simulink library "vehicle_dynamics_lib"  (R2012b)
settings: Solver=ode45  StartTime=0.0  StopTime=10.0  RelTol=1e-3
undefined symbols (not defined in the file): X, Y
settings Model: Creator=vismso  LastModifiedBy=vikafla

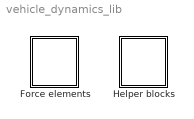
== system vehicle_dynamics_lib ==
  Force elements : Subsystem
  Helper blocks : Subsystem

== system vehicle_dynamics_lib/Force elements ==
  Spring-Damper : Subsystem  mask{dtype=Active, pdamp=on, c=[-1 1;-60.8e3 60.8e3], l0=0.253, d=[-1 1;-1.2e3 1.2e3], d_s_max=1200}
      mask prompts: dtype "Damper type"; pdamp "With passive damper?"; c "Spring stiffness table [displacement ...;force ...]"; l0 "Spring free length [m]"; d "Damper cushioning table [velocity ...;force ...]"; d_s_max "Maximum active damper damping value [Ns/m]"
      settings: MinAlgLoopOccurrences=on
      mask TypeOptions dtype: Semi-active | Active | Passive
      mask Callback dtype:
      | % set control visibilities
      | pdamp = get_param(gcb,'pdamp');
      | if strcmpi(get_param(gcb,'dtype'),'active')
      |     set_param(gcb,'MaskVisibilities',{'on','on','on','on',pdamp,'off'});
      |     set_param(gcb,'pdamp',pdamp);
      | elseif strcmpi(get_param(gcb,'dtype'),'passive')
      |     set_param(gcb,'MaskVisibilities',{'on','off','on','on','on','off'});
      |     set_param(gcb,'pdamp','on');
      | else
      |     set_param(gcb,'MaskVisibilities',{'on','off','on','on','off','on'});
      |     set_param(gcb,'pdamp','off');
      | end
      mask Callback pdamp:
      | tempvis = get_param(gcb,'MaskVisibilities');
      | if strcmpi(get_param(gcb,'pdamp'),'on')
      |     tempvis{5} = 'on';
      |     set_param(gcb,'MaskVisibilities',tempvis);
      | else
      |     tempvis{5} = 'off';
      |     set_param(gcb,'MaskVisibilities',tempvis);
      | end
      mask Display:
      | image(imread('damper.jpg'))
      | color('white')
      | port_label('input',2,'Actuator Force')
  Wheel forces & torques : Subsystem  mask{c=200e3, d=1e3, r0=0.24}
      mask prompts: c "Tire spring stiffness [N/m]"; d "Tire damper cushioning [N/(m/s)]"; r0 "Unloaded tire radius [m]"
      settings: MinAlgLoopOccurrences=on
      mask Display: image(imread('tire.jpg'))
  Wheel forces & torques (Pacejka stationary) : Subsystem  mask{c=200e3, d=1e3, r0=0.33, a=[1.799,0,1088,1140,6.026,0,-0.3589,1,0,-6.111e-3,-3.224e-2,0,0,0,0], b=[1.45,0,1088,0,129,0,0,0,-7,0,0]}
      mask prompts: c "Tire spring stiffness [N/m]"; d "Tire damper cushioning [N/(m/s)]"; r0 "Unloaded tire radius [m]"; a "Pacejka lateral a values (14)"; b "Pacejka longitudunal b values (10)"
      settings: MinAlgLoopOccurrences=on
      mask Display: image(imread('tire.jpg'))
  Wheel forces & torques (Pacejka transient) : Subsystem  mask{c=200e3, d=1e3, r0=0.33, a=[1.799,0,1088,1140,6.026,0,-0.3589,1,0,-6.111e-3,-3.224e-2,0,0,0,0], b=[1.45,0,1088,0,129,0,0,0,-7,0,0], Lx=0.2, Ly=0.2, Vlow=2}
      mask prompts: c "Tire spring stiffness [N/m]"; d "Tire damper cushioning [N/(m/s)]"; r0 "Unloaded tire radius [m]"; a "Pacejka lateral a values (15)"; b "Pacejka longitudunal b values (11)"; Lx "Longitudinal relaxation length [m]"; Ly "Lateral relaxation length [m]"; Vlow "Lower speed limit for slip damping [m/s]"
      settings: MinAlgLoopOccurrences=on
      mask Display: image(imread('tire.jpg'))

== system vehicle_dynamics_lib/Helper blocks ==
  2nd order butterworth high-pass : Subsystem  mask{wf=0.07, zeta=1/sqrt(2)}
      mask prompts: wf "Cut-off frequency [Hz]"; zeta "Damping coefficient"
      mask init:
      | x = 0:1:2;
      | y = [0;1;1];
      mask Display:
      | plot(x,y)
      | text(1,0.5,'HP')
  Lookup-table for ground geometry : Subsystem  mask(Lookup-table for ground geometry){}
      mask help:
      | This block contains the lookup tables holding data for the ground grid
      | lookup. It reads the variables X, Y, Z ,Nx , Ny, Nz from Matlabs
      | workspace. All of these variables must be meshgrids of equal size.
      |
      | X,Y - X,Y Positions
      | Z - Grid of ground height corresponding to X,Y values
      | Nx,Ny,Nz - Components of normal vector for each X,Y point of the ground
      |
      | Given input x,y coordinates, the block outputs the corresponding ground
      | height Z value and the points surface normal.
  Numerical differentiator : Subsystem  mask{Ts=0.01}
      mask prompts: Ts "First order lag time constant [s]"
      mask init:
      | x = 0:0.1:9;
      | y = exp(-x);
      mask Display:
      | plot(x,y)
      | text(3.5,0.5,'d/dt')
  "q1dot -> q" : Subsystem  mask(Euler angle -> Quaternion integration){}
      mask help:
      | This block internally integrates given euler angles as quaternions, thus
      | evading gimbal lock.
      mask Display: droots([],[0],1)

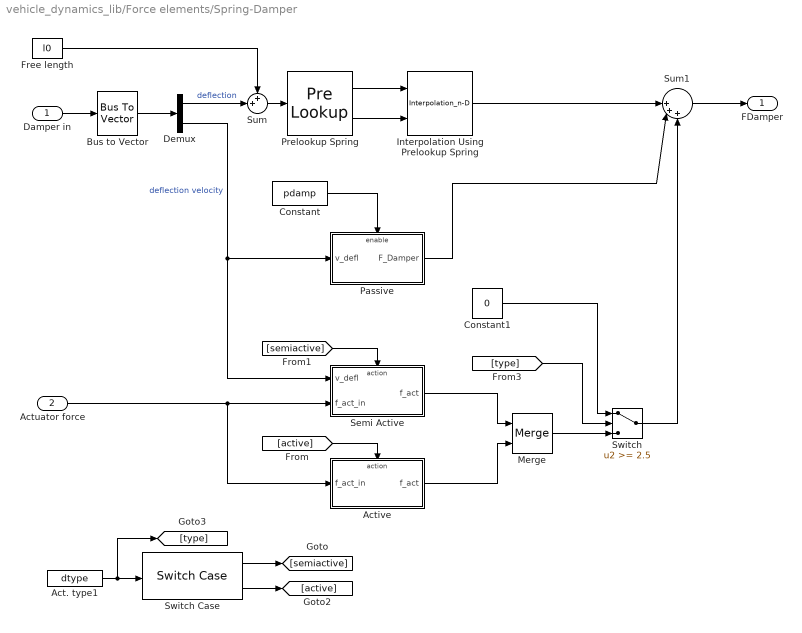
== system vehicle_dynamics_lib/Force elements/Spring-Damper ==
  Damper in : Inport
  Actuator force : Inport  Port=2
  Act. type1 : Constant  Value=dtype
      settings: AttributesFormatString=1 = semi-active\n2 = active\n3 = passive
  Active : Subsystem  TreatAsAtomicUnit=on
  Bus to Vector : BusToVector
  Constant : Constant  Value=pdamp
  Constant1 : Constant  Value=0
  Demux : Demux  Outputs=2
  Free length : Constant  Value=l0
  Interpolation Using Prelookup Spring : Interpolation_n-D  NumberOfTableDimensions=1  Table=c(2,:)
      settings: InputPortMap=u0,u1
  Merge : Merge
  Passive : Subsystem  TreatAsAtomicUnit=on
  Prelookup Spring : PreLookup  BreakpointsData=c(1,:)  ExtrapMethod=Linear
  Semi Active : Subsystem  TreatAsAtomicUnit=on
  Sum : Sum  Inputs=++|
  Sum1 : Sum  Inputs=||+++
  Switch : Switch  Threshold=2.5
  Switch Case : SwitchCase  CaseConditions={1,2}  ShowDefaultCase=off
  FDamper : Outport
  wires:
  Demux/2 -> Passive/1(v_defl), Semi Active/1(v_defl)  "deflection velocity"
  Demux/1 -> Sum/2  "deflection"
  Bus to Vector/1 -> Demux/1
  Interpolation Using Prelookup Spring/1 -> Sum1/1
  Sum1/1 -> FDamper/1
  Free length/1 -> Sum/1
  Damper in/1 -> Bus to Vector/1
  Sum/1 -> Prelookup Spring/1
  Prelookup Spring/2 -> Interpolation Using Prelookup Spring/2
  Prelookup Spring/1 -> Interpolation Using Prelookup Spring/1
  Act. type1/1 -> Switch Case/1, [type]
  Actuator force/1 -> Semi Active/2(f_act_in), Active/1(f_act_in)
  Switch Case/1 -> [semiactive]
  Switch Case/2 -> [active]
  [active] -> Active/Action
  [semiactive] -> Semi Active/Action
  [type] -> Switch/2
  Constant/1 -> Passive/Enable
  Passive/1(F_Damper) -> Sum1/2
  Active/1(f_act) -> Merge/2
  Semi Active/1(f_act) -> Merge/1
  Switch/1 -> Sum1/3
  Constant1/1 -> Switch/1
  Merge/1 -> Switch/3

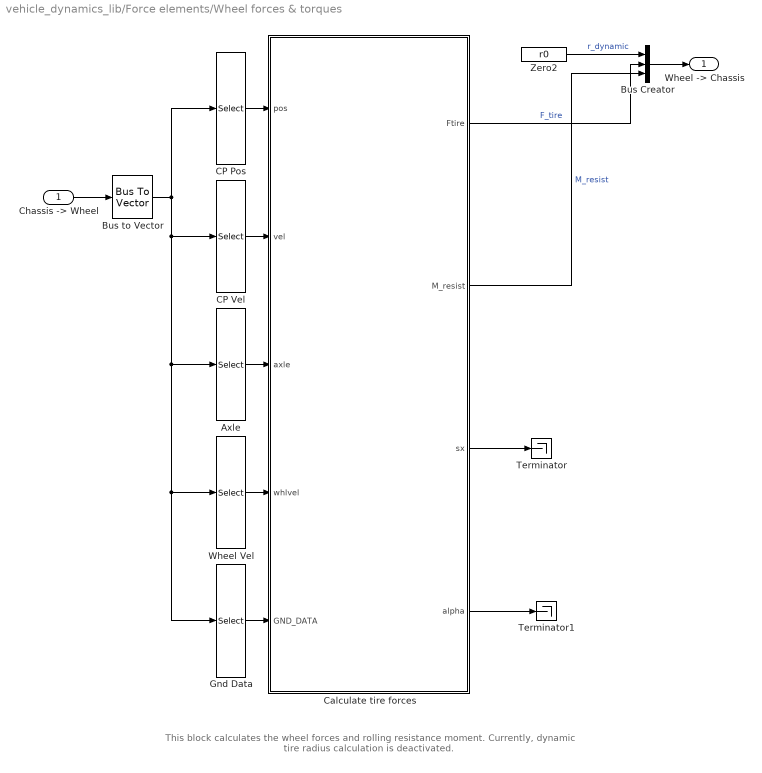
== system vehicle_dynamics_lib/Force elements/Wheel forces & torques ==
  note: This block calculates the wheel forces and rolling resistance moment.
      | Currently, dynamic tire radius calculation is deactivated.
  "Chassis -> Wheel" : Inport
  Axle : Selector  InputPortWidth=16  IndexOptions=Index vector (dialog)  Indices=[1:3]  OutputSizes=1
  Bus Creator : BusCreator  Inputs=3
  Bus to Vector : BusToVector
  CP Pos : Selector  InputPortWidth=16  IndexOptions=Index vector (dialog)  Indices=[4:6]  OutputSizes=1
  CP Vel : Selector  InputPortWidth=16  IndexOptions=Index vector (dialog)  Indices=[7:9]  OutputSizes=1
  Calculate tire forces : MATLAB Function  TreatAsAtomicUnit=on
  Gnd Data : Selector  InputPortWidth=16  IndexOptions=Index vector (dialog)  Indices=[13:16]  OutputSizes=1
  Terminator : Terminator
  Terminator1 : Terminator
  Wheel Vel : Selector  InputPortWidth=16  IndexOptions=Index vector (dialog)  Indices=[10:12]  OutputSizes=1
  Zero2 : Constant  Value=r0
  "Wheel -> Chassis" : Outport
  wires:
  Gnd Data/1 -> Calculate tire forces/5(GND_DATA)
  Calculate tire forces/4(alpha) -> Terminator1/1
  Calculate tire forces/3(sx) -> Terminator/1
  Bus Creator/1 -> "Wheel -> Chassis"/1
  Calculate tire forces/2(M_resist) -> Bus Creator/3  "M_resist"
  Zero2/1 -> Bus Creator/1  "r_dynamic"
  CP Pos/1 -> Calculate tire forces/1(pos)
  CP Vel/1 -> Calculate tire forces/2(vel)
  Calculate tire forces/1(Ftire) -> Bus Creator/2  "F_tire"
  "Chassis -> Wheel"/1 -> Bus to Vector/1
  Bus to Vector/1 -> CP Pos/1, CP Vel/1, Gnd Data/1, Wheel Vel/1, Axle/1
  Axle/1 -> Calculate tire forces/3(axle)
  Wheel Vel/1 -> Calculate tire forces/4(whlvel)

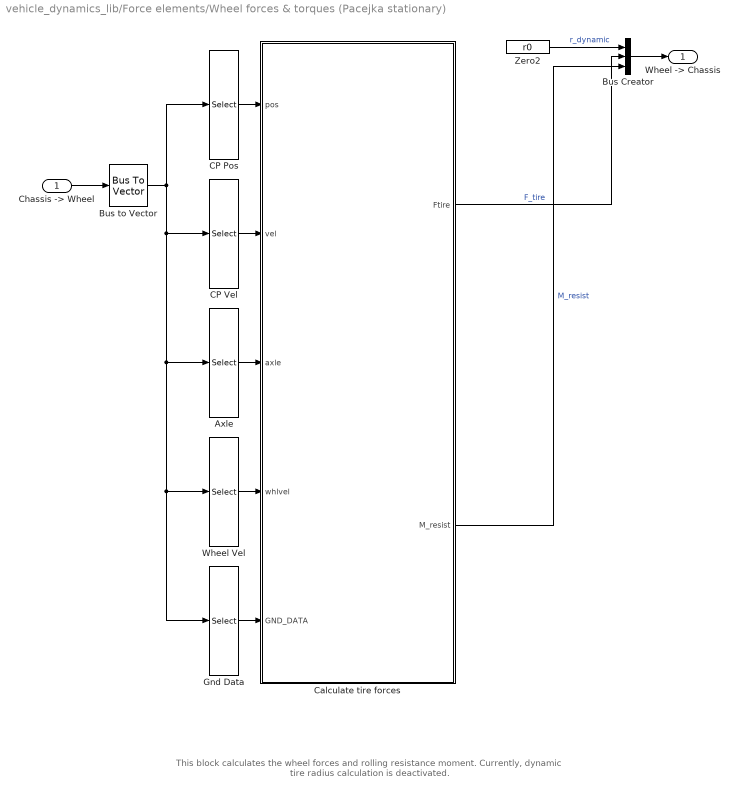
== system vehicle_dynamics_lib/Force elements/Wheel forces & torques (Pacejka stationary) ==
  note: This block calculates the wheel forces and rolling resistance moment.
      | Currently, dynamic tire radius calculation is deactivated.
  "Chassis -> Wheel" : Inport
  Axle : Selector  InputPortWidth=16  IndexOptions=Index vector (dialog)  Indices=[1:3]  OutputSizes=1
  Bus Creator : BusCreator  Inputs=3
  Bus to Vector : BusToVector
  CP Pos : Selector  InputPortWidth=16  IndexOptions=Index vector (dialog)  Indices=[4:6]  OutputSizes=1
  CP Vel : Selector  InputPortWidth=16  IndexOptions=Index vector (dialog)  Indices=[7:9]  OutputSizes=1
  Calculate tire forces : MATLAB Function  TreatAsAtomicUnit=on
  Gnd Data : Selector  InputPortWidth=16  IndexOptions=Index vector (dialog)  Indices=[13:16]  OutputSizes=1
  Wheel Vel : Selector  InputPortWidth=16  IndexOptions=Index vector (dialog)  Indices=[10:12]  OutputSizes=1
  Zero2 : Constant  Value=r0
  "Wheel -> Chassis" : Outport
  wires:
  Gnd Data/1 -> Calculate tire forces/5(GND_DATA)
  Bus Creator/1 -> "Wheel -> Chassis"/1
  Calculate tire forces/2(M_resist) -> Bus Creator/3  "M_resist"
  Zero2/1 -> Bus Creator/1  "r_dynamic"
  CP Pos/1 -> Calculate tire forces/1(pos)
  CP Vel/1 -> Calculate tire forces/2(vel)
  Calculate tire forces/1(Ftire) -> Bus Creator/2  "F_tire"
  "Chassis -> Wheel"/1 -> Bus to Vector/1
  Bus to Vector/1 -> CP Pos/1, CP Vel/1, Gnd Data/1, Wheel Vel/1, Axle/1
  Axle/1 -> Calculate tire forces/3(axle)
  Wheel Vel/1 -> Calculate tire forces/4(whlvel)

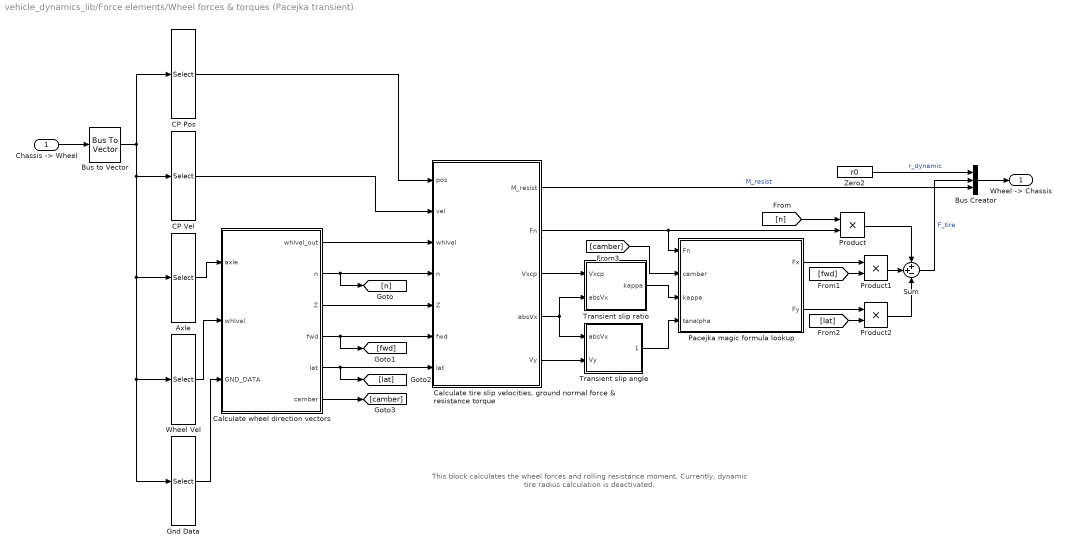
== system vehicle_dynamics_lib/Force elements/Wheel forces & torques (Pacejka transient) ==
  note: This block calculates the wheel forces and rolling resistance moment.
      | Currently, dynamic tire radius calculation is deactivated.
  "Chassis -> Wheel" : Inport
  Axle : Selector  InputPortWidth=16  IndexOptions=Index vector (dialog)  Indices=[1:3]  OutputSizes=1
  Bus Creator : BusCreator  Inputs=3
  Bus to Vector : BusToVector
  CP Pos : Selector  InputPortWidth=16  IndexOptions=Index vector (dialog)  Indices=[4:6]  OutputSizes=1
  CP Vel : Selector  InputPortWidth=16  IndexOptions=Index vector (dialog)  Indices=[7:9]  OutputSizes=1
  "Calculate tire slip velocities, ground normal force & resistance torque" : MATLAB Function  TreatAsAtomicUnit=on
  Calculate wheel direction vectors : MATLAB Function  TreatAsAtomicUnit=on
  Gnd Data : Selector  InputPortWidth=16  IndexOptions=Index vector (dialog)  Indices=[13:16]  OutputSizes=1
  Pacejka magic formula lookup : MATLAB Function  TreatAsAtomicUnit=on
  Product : Product  RndMeth=Zero
  Product1 : Product  RndMeth=Zero
  Product2 : Product  RndMeth=Zero
  Sum : Sum  Inputs=++-
  Transient slip angle : Subsystem
  Transient slip ratio : Subsystem
  Wheel Vel : Selector  InputPortWidth=16  IndexOptions=Index vector (dialog)  Indices=[10:12]  OutputSizes=1
  Zero2 : Constant  Value=r0
  "Wheel -> Chassis" : Outport
  wires:
  Bus to Vector/1 -> Axle/1, Wheel Vel/1, Gnd Data/1, CP Vel/1, CP Pos/1
  "Chassis -> Wheel"/1 -> Bus to Vector/1
  Sum/1 -> Bus Creator/2  "F_tire"
  CP Pos/1 -> "Calculate tire slip velocities, ground normal force & resistance torque"/1(pos)
  Zero2/1 -> Bus Creator/1  "r_dynamic"
  Bus Creator/1 -> "Wheel -> Chassis"/1
  CP Vel/1 -> "Calculate tire slip velocities, ground normal force & resistance torque"/2(vel)
  "Calculate tire slip velocities, ground normal force & resistance torque"/3(Vxcp) -> Transient slip ratio/1(Vxcp)
  "Calculate tire slip velocities, ground normal force & resistance torque"/4(absVx) -> Transient slip ratio/2(absVx), Transient slip angle/1(absVx)
  "Calculate tire slip velocities, ground normal force & resistance torque"/5(Vy) -> Transient slip angle/2(Vy)
  "Calculate tire slip velocities, ground normal force & resistance torque"/2(Fn) -> Pacejka magic formula lookup/1(Fn), Product/2
  Transient slip ratio/1(kappa) -> Pacejka magic formula lookup/3(kappa)
  Transient slip angle/1(tanalpha) -> Pacejka magic formula lookup/4(tanalpha)
  Axle/1 -> Calculate wheel direction vectors/1(axle)
  Wheel Vel/1 -> Calculate wheel direction vectors/2(whlvel)
  Gnd Data/1 -> Calculate wheel direction vectors/3(GND_DATA)
  Calculate wheel direction vectors/2(n) -> "Calculate tire slip velocities, ground normal force & resistance torque"/4(n), [n]
  Calculate wheel direction vectors/3(Z) -> "Calculate tire slip velocities, ground normal force & resistance torque"/5(Z)
  Calculate wheel direction vectors/4(fwd) -> "Calculate tire slip velocities, ground normal force & resistance torque"/6(fwd), [fwd]
  Calculate wheel direction vectors/5(lat) -> "Calculate tire slip velocities, ground normal force & resistance torque"/7(lat), [lat]
  Calculate wheel direction vectors/1(whlvel_out) -> "Calculate tire slip velocities, ground normal force & resistance torque"/3(whlvel)
  "Calculate tire slip velocities, ground normal force & resistance torque"/1(M_resist) -> Bus Creator/3  "M_resist"
  Product/1 -> Sum/1
  [n] -> Product/1
  Product1/1 -> Sum/2
  Pacejka magic formula lookup/1(Fx) -> Product1/1
  [fwd] -> Product1/2
  Pacejka magic formula lookup/2(Fy) -> Product2/1
  [lat] -> Product2/2
  Product2/1 -> Sum/3
  Calculate wheel direction vectors/6(camber) -> [camber]
  [camber] -> Pacejka magic formula lookup/2(camber)

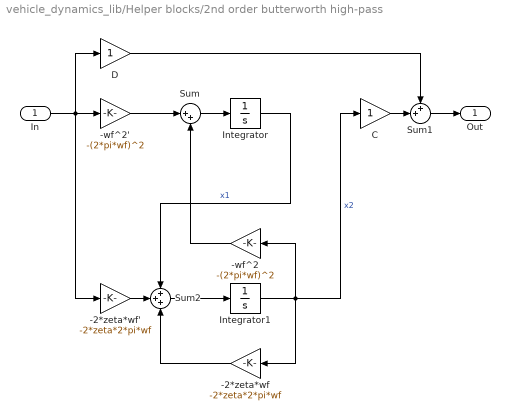
== system vehicle_dynamics_lib/Helper blocks/2nd order butterworth high-pass ==
  In : Inport
  -2*zeta*wf : Gain  Gain=-2*zeta*2*pi*wf
  -2*zeta*wf' : Gain  Gain=-2*zeta*2*pi*wf
  -wf^2 : Gain  Gain=-(2*pi*wf)^2
  -wf^2' : Gain  Gain=-(2*pi*wf)^2
  C : Gain
  D : Gain
  Integrator : Integrator
  Integrator1 : Integrator
  Sum : Sum  Inputs=|++
  Sum1 : Sum  Inputs=++|
  Sum2 : Sum  Inputs=+++
  Out : Outport
  wires:
  D/1 -> Sum1/1
  C/1 -> Sum1/2
  Integrator/1 -> Sum2/1  "x1"
  -wf^2'/1 -> Sum/1
  In/1 -> -wf^2'/1, D/1, -2*zeta*wf'/1
  Sum/1 -> Integrator/1
  Integrator1/1 -> -wf^2/1, -2*zeta*wf/1, C/1  "x2"
  Sum2/1 -> Integrator1/1
  -wf^2/1 -> Sum/2
  -2*zeta*wf/1 -> Sum2/3
  -2*zeta*wf'/1 -> Sum2/2
  Sum1/1 -> Out/1

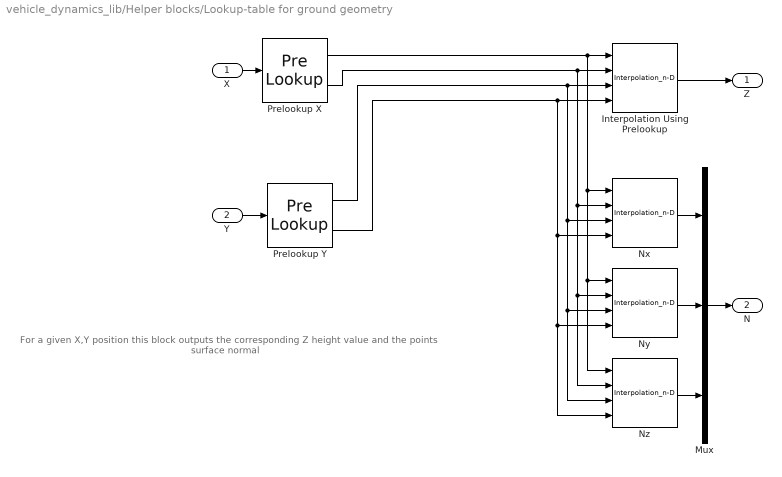
== system vehicle_dynamics_lib/Helper blocks/Lookup-table for ground geometry ==
  note: For a given X,Y position this block outputs the
      | corresponding Z height value and the points surface normal
  X : Inport
  Y : Inport  Port=2
  Interpolation Using Prelookup : Interpolation_n-D  Table=Z.'  RemoveProtectionIndex=on  TableDataTypeStr=Inherit: Inherit from 'Table data'
  Mux : Mux  Inputs=3
  Nx : Interpolation_n-D  Table=Nx.'  ExtrapMethod=Clip  RemoveProtectionIndex=on  TableDataTypeStr=Inherit: Inherit from 'Table data'
  Ny : Interpolation_n-D  Table=Ny.'  ExtrapMethod=Clip  RemoveProtectionIndex=on  TableDataTypeStr=Inherit: Inherit from 'Table data'
  Nz : Interpolation_n-D  Table=Nz.'  ExtrapMethod=Clip  RemoveProtectionIndex=on  TableDataTypeStr=Inherit: Inherit from 'Table data'
  Prelookup X : PreLookup  BreakpointsData=X(1,:)  ExtrapMethod=Linear  BreakpointDataTypeStr=Inherit: Inherit from 'Breakpoint data'
  Prelookup Y : PreLookup  BreakpointsData=Y(:,1)  ExtrapMethod=Linear  BreakpointDataTypeStr=Inherit: Inherit from 'Breakpoint data'
  Z : Outport
  N : Outport  Port=2  PortDimensions=3
  wires:
  Mux/1 -> N/1
  Prelookup X/2 -> Interpolation Using Prelookup/2, Nz/2, Ny/2, Nx/2
  Prelookup X/1 -> Interpolation Using Prelookup/1, Ny/1, Nz/1, Nx/1
  Prelookup Y/2 -> Interpolation Using Prelookup/4, Nz/4, Ny/4, Nx/4
  Prelookup Y/1 -> Interpolation Using Prelookup/3, Nz/3, Ny/3, Nx/3
  Nz/1 -> Mux/3
  Ny/1 -> Mux/2
  Y/1 -> Prelookup Y/1
  Nx/1 -> Mux/1
  Interpolation Using Prelookup/1 -> Z/1
  X/1 -> Prelookup X/1

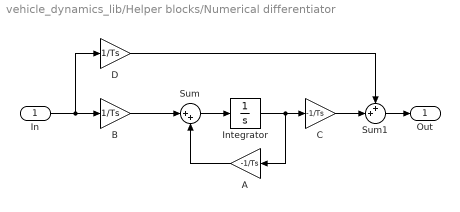
== system vehicle_dynamics_lib/Helper blocks/Numerical differentiator ==
  In : Inport
  A : Gain  Gain=-1/Ts
  B : Gain  Gain=1/Ts
  C : Gain  Gain=-1/Ts
  D : Gain  Gain=1/Ts
  Integrator : Integrator
  Sum : Sum  Inputs=|++
  Sum1 : Sum  Inputs=++|
  Out : Outport
  wires:
  Sum/1 -> Integrator/1
  In/1 -> B/1, D/1
  B/1 -> Sum/1
  Integrator/1 -> A/1, C/1
  A/1 -> Sum/2
  C/1 -> Sum1/2
  D/1 -> Sum1/1
  Sum1/1 -> Out/1

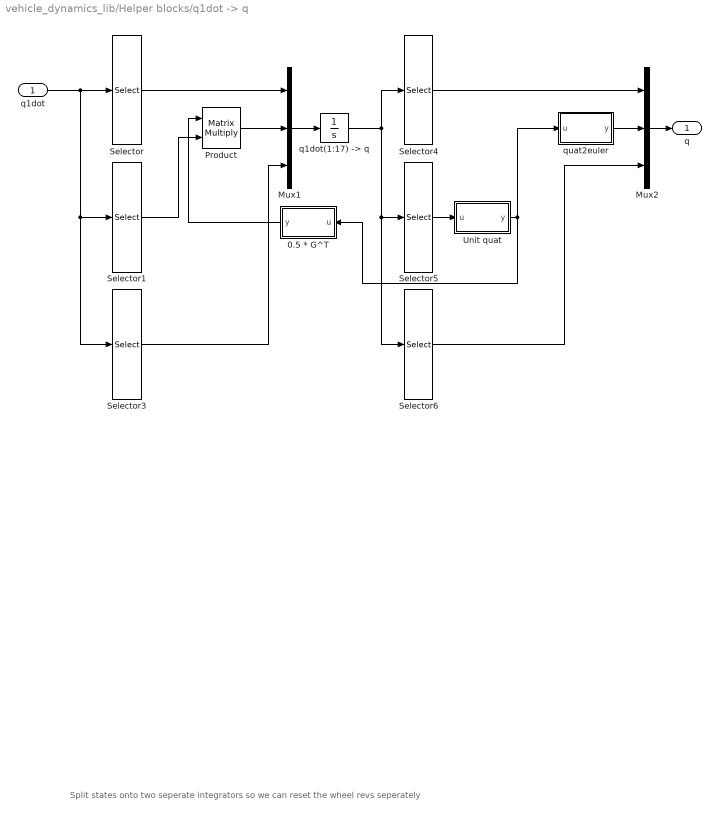
== system vehicle_dynamics_lib/Helper blocks/q1dot -> q ==
  note: Split states onto two seperate integrators so we can reset the wheel revs seperately
  q1dot : Inport
  0.5 * G^T : MATLAB Function  TreatAsAtomicUnit=on
  Mux1 : Mux  Inputs=3
  Mux2 : Mux  Inputs=3
  Product : Product  Multiplication=Matrix(*)  RndMeth=Zero
  Selector : Selector  InputPortWidth=16  IndexOptions=Index vector (dialog)  Indices=[1:3]  OutputSizes=1
  Selector1 : Selector  InputPortWidth=16  IndexOptions=Index vector (dialog)  Indices=[4:6]  OutputSizes=1
  Selector3 : Selector  InputPortWidth=16  IndexOptions=Index vector (dialog)  Indices=[7:16]  OutputSizes=1
  Selector4 : Selector  InputPortWidth=17  IndexOptions=Index vector (dialog)  Indices=[1:3]  OutputSizes=1
  Selector5 : Selector  InputPortWidth=17  IndexOptions=Index vector (dialog)  Indices=[4:7]  OutputSizes=1
  Selector6 : Selector  InputPortWidth=17  IndexOptions=Index vector (dialog)  Indices=[8:17]  OutputSizes=1
  Unit quat : MATLAB Function  TreatAsAtomicUnit=on
  "q1dot(1:17) -> q" : Integrator  InitialCondition=[0;0;2;1;0;0;0;zeros(10,1)]
  quat2euler : MATLAB Function  TreatAsAtomicUnit=on
  q : Outport
  wires:
  Unit quat/1(y) -> 0.5 * G^T/1(u), quat2euler/1(u)
  "q1dot(1:17) -> q"/1 -> Selector6/1, Selector5/1, Selector4/1
  Selector6/1 -> Mux2/3
  quat2euler/1(y) -> Mux2/2
  Selector5/1 -> Unit quat/1(u)
  Selector4/1 -> Mux2/1
  Mux2/1 -> q/1
  Selector3/1 -> Mux1/3
  Product/1 -> Mux1/2
  Selector/1 -> Mux1/1
  Mux1/1 -> "q1dot(1:17) -> q"/1
  Selector1/1 -> Product/2
  0.5 * G^T/1(y) -> Product/1
  q1dot/1 -> Selector3/1, Selector1/1, Selector/1

== system vehicle_dynamics_lib/Force elements/Spring-Damper/Active ==
  f_act_in : Inport
  Action Port : ActionPort  ActionType=case
  f_act : Outport
  wires:
  f_act_in/1 -> f_act/1

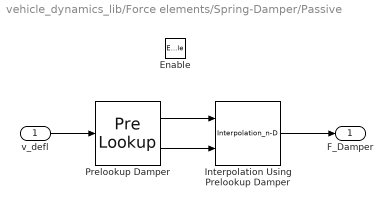
== system vehicle_dynamics_lib/Force elements/Spring-Damper/Passive ==
  v_defl : Inport
  Enable : EnablePort  StatesWhenEnabling=reset
  Interpolation Using Prelookup Damper : Interpolation_n-D  NumberOfTableDimensions=1  Table=d(2,:)
      settings: InputPortMap=u0,u1
  Prelookup Damper : PreLookup  BreakpointsData=d(1,:)  ExtrapMethod=Linear
  F_Damper : Outport  OutputWhenDisabled=reset  InitialOutput=0
  wires:
  Prelookup Damper/2 -> Interpolation Using Prelookup Damper/2
  Prelookup Damper/1 -> Interpolation Using Prelookup Damper/1
  v_defl/1 -> Prelookup Damper/1
  Interpolation Using Prelookup Damper/1 -> F_Damper/1

== system vehicle_dynamics_lib/Force elements/Spring-Damper/Semi Active ==
  v_defl : Inport
  f_act_in : Inport  Port=2
  Action Port : ActionPort  ActionType=case
  Semi-active force : MATLAB Function  TreatAsAtomicUnit=on
  f_act : Outport
  wires:
  Semi-active force/1(f_out) -> f_act/1
  f_act_in/1 -> Semi-active force/2(f_in)
  v_defl/1 -> Semi-active force/1(v_defl)

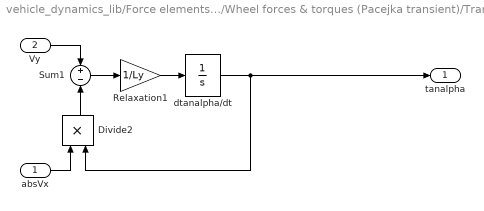
== system vehicle_dynamics_lib/Force elements/Wheel forces & torques (Pacejka transient)/Transient slip angle ==
  absVx : Inport
  Vy : Inport  Port=2
  Divide2 : Product
  Relaxation1 : Gain  Gain=1/Ly
  Sum1 : Sum  Inputs=+-
  dtanalpha/dt : Integrator
  tanalpha : Outport
  wires:
  Relaxation1/1 -> dtanalpha/dt/1
  Sum1/1 -> Relaxation1/1
  Divide2/1 -> Sum1/2
  dtanalpha/dt/1 -> Divide2/2, tanalpha/1
  Vy/1 -> Sum1/1
  absVx/1 -> Divide2/1

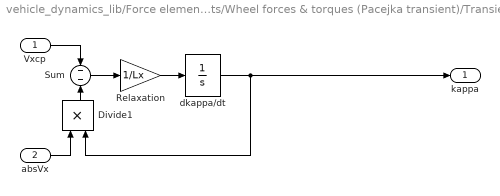
== system vehicle_dynamics_lib/Force elements/Wheel forces & torques (Pacejka transient)/Transient slip ratio ==
  Vxcp : Inport
  absVx : Inport  Port=2
  Divide1 : Product
  Relaxation : Gain  Gain=1/Lx
  Sum : Sum  Inputs=--
  dkappa/dt : Integrator
  kappa : Outport
  wires:
  Relaxation/1 -> dkappa/dt/1
  Sum/1 -> Relaxation/1
  Divide1/1 -> Sum/2
  dkappa/dt/1 -> Divide1/2, kappa/1
  absVx/1 -> Divide1/1
  Vxcp/1 -> Sum/1

== matlab function vehicle_dynamics_lib/Helper blocks/q1dot -> q/0.5 * G^T ==
  data: u input; y output
function y = fcn(u)
%#eml
e = u(2:4);
etilde = [0,-u(4),u(3);u(4),0,-u(2);-u(3),u(2),0];
e0 = u(1);

G = [-e etilde+e0*eye(3)];

y = 0.5*G.';

== matlab function vehicle_dynamics_lib/Force elements/Wheel forces & torques (Pacejka transient)/Calculate wheel direction vectors ==
  data: whlvel_out output size=3; n output size=3; Z output size=1; fwd output size=3; lat output size=3; axle input size=3; whlvel input size=3; GND_DATA input size=4; camber output
function [whlvel_out, n, Z, fwd, lat, camber] = tire_vectors(axle, whlvel, GND_DATA)
%#eml

n = GND_DATA(2:4);    % Normal to ground
Z = GND_DATA(1);    % z-height of ground


fwd = cross(axle,n);        % forward direction vector
fwd_len = sqrt(fwd.'*fwd);
if( fwd_len < 1e-6 )
	% wheel axle nearly orthogonal to ground normal   
	whlvel_out = [0;0;0];
else
	whlvel_out = whlvel;
end
fwd = fwd/fwd_len;  % longitudinal unit vector

lat = cross(n,fwd);  % lateral unit vector

camber = 0;         % TODO: camber calculation NYI

== matlab function vehicle_dynamics_lib/Helper blocks/q1dot -> q/quat2euler ==
  data: u input; y output
function y = fcn(u)
%#eml
sqw = u(1)*u(1);
sqx = u(2)*u(2);
sqy = u(3)*u(3);
sqz = u(4)*u(4);

unit = sqx + sqy + sqz + sqw;
test = u(2)*u(4) + u(1)*u(3);
if (test > 0.495*unit)
    heading = 2 * atan2(u(2),u(1));
	attitude = pi/2;
	bank = 0;
elseif (test < -0.495*unit)
	heading = -2 * atan2(u(2),u(1));
	attitude = -pi/2;
	bank = 0;
else
    heading = atan2(2*(u(1)*u(2)-u(3)*u(4)) , sqw - sqx -sqy +sqz);
	attitude = asin(2*test);
	bank = atan2(2*(u(1)*u(4)-u(2)*u(3)) , sqw+sqx-sqy-sqz);
end

y=[heading;attitude;bank];
%y = [
%atan2(2*(u(1)*u(2)+u(3)*u(4)),1-2*(u(2)^2+u(3)^2));
%asin(2*(u(1)*u(3)-u(4)*u(2)));
%atan2(2*(u(1)*u(4)+u(2)*u(3)),1-2*(u(3)^2+u(4)^2))
%];

== matlab function vehicle_dynamics_lib/Helper blocks/q1dot -> q/Unit quat ==
  data: u input; y output
function y = fcn(u)
%#eml

y = u/sqrt(u.'*u);

== matlab function vehicle_dynamics_lib/Force elements/Wheel forces & torques (Pacejka stationary)/Calculate tire forces ==
  data: pos input size=3; Ftire output size=3; M_resist output; vel input size=3; axle input size=3; whlvel input size=3; GND_DATA input; c parameter size=1; d parameter size=1; r0 parameter; a parameter size=15; b parameter size=11
function [Ftire, M_resist] = tire_force(pos, vel, axle, whlvel, GND_DATA , c, d, r0, a, b)
%#eml
persistent last_whlvel_x; if isempty(last_whlvel_x), last_whlvel_x = 0; end

n = GND_DATA(2:4);    % Normal to ground
Z = GND_DATA(1);    % z-height of ground
v_thres = 1e-1; % Threshold of slip
mu = 1;          % road friciton coefficient
qsy1 = 0.01;    % rolling friction coefficient
V0 = 16.66;     % reference velocity [m/s]
B = 0.2;       % relaxation length [m]

%% Calculate normal force
defl_n = n.'*([0;0;pos(3)-Z]);
if defl_n > 0   % No forces if wheel doesn't touch ground
    Ftire = zeros(3,1);
    M_resist = 0;
    return;
end

Fn = -c*defl_n; % Vertical force due to tire stiffness
vel_n = n.'*vel;  % velocity of contact point normal to ground

if vel_n < 0    % damper only generates force on contraction
    Fn=Fn-d*vel_n;  
end

%% Calculate slip & slip angle
fwd = cross(axle,n);        % forward direction vector
fwd_len = sqrt(fwd.'*fwd);
%if( fwd_len < 1e-6 )
%   wheel axle nearly orthogonal to ground normal   
%end
fwd = fwd/fwd_len;  % longitudinal unit vector

lat = cross(n,fwd);  % lateral unit vector

camber = 0; %acos(axle.'*n)-pi/2;

% x-Dir
vx = fwd.'*vel;
whlvel_x = fwd.'*whlvel;
awhlvel_x = abs(whlvel_x);

if( whlvel_x*0.005/B>0.5 )
    sx = vx/(whlvel_x);
else
    sx = vx/(whlvel_x+v_thres);
end

tmp = tanh(sqrt(vx*vx)/v_thres);
sx = tmp*tmp*sx;

if( sign(last_whlvel_x)*sign(whlvel_x) < 0 )
    sx = -0.1*sx;
end 
last_whlvel_x = whlvel_x;


% y-Dir
whlvel_y = lat.'*whlvel;
%tmp = tanh(sqrt(whlvel_x*whlvel_x + whlvel_y*whlvel_y)/alpha_thres); % reduce alpha for low speeds
%alpha = abs(alpha*tmp*tmp);
if( abs(whlvel.'*fwd) < v_thres || abs(whlvel.'*lat) < v_thres )
    alpha = 0;
else
    alpha = atan2(whlvel_y,awhlvel_x);
end


[Fx, Fy] = pacejka(Fn, mu, sx, alpha, camber, a, b);

Ftire = n*Fn - fwd*Fx - lat*Fy;
fr = qsy1;
Fr = fr*Fn; % free rolling resistance
M_resist = -Fr*r0*tanh((whlvel_x-vx)/V0);
%% Calculate friction torque

function [Fx, Fy ] = pacejka( Fz, mu, sx, alpha, camber, a, b )
%TIRE_FORCE(Fz, mu, sx, alpha)
%   Calculation of lateral and longitudinal tire forces 
%       <Vehicle Dynamics, p. 48>
%   Fz - vertical load force in N
%   mu - road-tire friction coefficient
%   sx - longitudinal slip
%   alpha - slip angle
Fz = Fz/1e3;    % Fz unit is kN
    
d3_eps = 1e-5;

slipPercentage = 100*sx;
sideSlip = alpha/pi*180;

FzSquared=Fz*Fz;
C=b(1);
uP=b(2)*Fz+b(3);
D=uP*Fz;
  
if( abs(C) < d3_eps || abs(D) < d3_eps )
	B=99999;
else
	B=((b(4)*FzSquared+b(5)*Fz)*exp(-b(6)*Fz))/(C*D);
end
  
E=b(7)*FzSquared+b(8)*Fz+b(9);
Sh=b(10)*Fz+b(11);
Sv=0;
  
% Notice that product BCD is the longitudinal tire stiffness
longStiffness=B*C*D;
  
% Remember the max longitudinal force (where sin(...)==1)
maxForce_x=(D+Sv)*mu;

% Calculate result force
Fx=(D*sin(C*atan(B*(1-E)*(slipPercentage+Sh)+ ...
      E*atan(B*(slipPercentage+Sh))))+Sv)*mu;

% Calculate derived coefficients
C=a(1);
uP=a(2)*Fz+a(3);
D=uP*Fz;
E=a(7)*Fz+a(8);
  
% Avoid div by 0
if( abs(C) < d3_eps || abs(D) < d3_eps )
	B=99999;
else
	if( abs(a(5)) < d3_eps )
		B=99999;
    else
        % Notice that product BCD is the lateral stiffness (=cornering)
        latStiffness=a(4)*sin(2*atan(Fz/a(5)))*(1-a(6)*abs(camber));
        B=latStiffness/(C*D);
	end
end

Sh=a(9)*camber+a(10)*Fz+a(11);
Sv=(a(12)*Fz+a(13))*camber*Fz+a(13)*Fz+a(14);
  
% Remember maximum lateral force
maxForce_y=(D+Sv)*mu;
  
% Calculate result force
Fy=(D*sin(C*atan(B*(1-E)*(sideSlip+Sh)+ ...
            E*atan(B*(sideSlip+Sh))))+Sv)*mu;
        
    
% Normalize the forces
if( abs(maxForce_y) < d3_eps || abs(maxForce_x) < d3_eps )
    return;
end

nrmFx=Fx/maxForce_x;
nrmFy=Fy/maxForce_y;

% Calculate total vector size, but avoid the sqrt() for now
len=nrmFy*nrmFy+nrmFx*nrmFx;
%{ 
If the vector exceeds the friction circle (which, because
it is normalized, is a real circle with radius 1), the
forces are downsized accordingly to fit the circle.
Note that 1 squared is still 1 (len is still squared)
%}
if( len > 1 )
	% Get actual length (non-squared)
    len=sqrt(len);

    Fx=Fx/len;
    Fy=Fy/len;
end

== matlab function vehicle_dynamics_lib/Force elements/Wheel forces & torques (Pacejka transient)/Calculate tire slip velocities, ground normal force & resistance torque ==
  data: M_resist output size=1; Fn output size=1; pos input size=3; Vxcp output size=1; absVx output size=1; Vy output size=1; vel input size=3; whlvel input size=3; n input size=3; Z input size=1; fwd input size=3; lat input size=3; c parameter size=1; d parameter size=1; r0 parameter size=1; Vlow parameter
function [M_resist, Fn, Vxcp, absVx, Vy] = tire_status(pos, vel, whlvel, n, Z, fwd, lat, c, d, r0, Vlow)
%#eml

qsy1 = 0.01;    % rolling friction coefficient
V0 = 16.66;     % reference velocity [m/s]

%% Calculate normal force
defl_n = n.'*([0;0;pos(3)-Z]);
if defl_n > 0   % No forces if wheel doesn't touch ground
    Vxcp = 0;
    Vy = 0;
    absVx = 0;
    M_resist = 0;
    Fn = 0;
    return;
end

Fn = -c*defl_n; % Vertical force due to tire stiffness
vel_n = n.'*vel;  % velocity of contact point normal to ground

if vel_n < 0    % damper only generates force on contraction
    Fn=Fn-d*vel_n;  
end

% x-Dir
Vxcp = fwd.'*vel;
Vx = fwd.'*whlvel;
if( Vx > Vlow )
	absVx = Vx;
elseif( Vx < -Vlow )
	absVx = -Vx;
else
    absVx = (Vx*Vx/Vlow+Vlow)/2;
end


% y-Dir
Vy = lat.'*whlvel;

fr = qsy1;
Fr = fr*Fn; % free rolling resistance
M_resist = -Fr*r0*tanh((Vx-Vxcp)/V0);

== matlab function vehicle_dynamics_lib/Force elements/Wheel forces & torques (Pacejka transient)/Pacejka magic formula lookup ==
  data: Fn input size=1; camber input; Fx output size=1; Fy output size=1; kappa input size=1; tanalpha input size=1; a parameter size=15; b parameter size=11
function [Fx, Fy] = pacejka_force(Fn,camber,kappa,tanalpha,a,b)
%#eml
%PACEJKA_FORCE(Fn, kappa, tanalpha, a,b)
%   Calculation of lateral and longitudinal tire forces 
%       <Vehicle Dynamics, p. 43>
%   Fn       - vertical load force in N
%   camber   - camber angle in radians
%   kappa    - slip
%   tanalpha - tangens of slip angle
%   a,b      - Pacejka parameters (a=lateral, b=longitudinal)

mu = 1;         % Friction coefficient (TODO: include in GND model)
d3_eps = 1e-5;

% --- Used for calculation of combined forces
kappaMax = 5;
alphaMax = 2.3;

kappa = 100*kappa;
kappaNrm = kappa/kappaMax;

alpha = atan(tanalpha)/pi*180;
alphaNrm = alpha/alphaMax;

rho = sqrt(kappaNrm^2+alphaNrm^2);

if( rho < d3_eps )
    rho = 1;
end
% ---

% --- Calculate separate lat & long forces
Fx = pacejka_Fx(Fn,rho*kappaMax,b);
Fy = pacejka_Fy(Fn,camber,rho*alphaMax,a);
% ---    
    
% --- Combine forces
Fx = kappaNrm/rho*Fx*mu;
Fy = alphaNrm/rho*Fy*mu;
% ---


%=%=%=%=%=%=%=%=%=%=%=%=%=%=%=%=%=%=%=%=%=%=%=%=%=%=%=%=%=%=%=%=%=%=%=%=%=%
%=%=% PACEJKA_FX                                                      %=%=%
%=%=%=%=%=%=%=%=%=%=%=%=%=%=%=%=%=%=%=%=%=%=%=%=%=%=%=%=%=%=%=%=%=%=%=%=%=%
function Fx = pacejka_Fx(Fn,kappa,b)
%#eml

Fz = Fn/1e3;    % Fz in kN
Fz2=Fz*Fz;
calc_eps = 1e-5;

%-- peak coefficient of friction
muP=b(2)*Fz+b(3);

%-- Calculate pacejka coefficients
% C
C=b(1);
% D
D=muP*Fz;
% B - Avoid division by zero
if( abs(C) < calc_eps || abs(D) < calc_eps )
	B=99999;
else
	B=((b(4)*Fz2+b(5)*Fz)*exp(-b(6)*Fz))/(C*D);
end
% E
E=b(7)*Fz2+b(8)*Fz+b(9);

% S = f(kappa)
S=kappa+b(10)*Fz+b(11);

% Resulting force
Fx=D*sin(C*atan(B*S-E*(B*S-atan(B*S))));

%=%=%=%=%=%=%=%=%=%=%=%=%=%=%=%=%=%=%=%=%=%=%=%=%=%=%=%=%=%=%=%=%=%=%=%=%=%
%=%=% PACEJKA_FY                                                      %=%=%
%=%=%=%=%=%=%=%=%=%=%=%=%=%=%=%=%=%=%=%=%=%=%=%=%=%=%=%=%=%=%=%=%=%=%=%=%=%
function Fy = pacejka_Fy(Fn,camber,alpha,a)
%#eml

Fz = Fn/1e3;    % Fz in kN
calc_eps = 1e-5;

%-- peak coefficient of friction
muP=a(2)*Fz+a(3);

%-- Calculate pacejka coefficients
% C
C=a(1);
% D
D=muP*Fz;
% B - Avoid division by 0
if( abs(C) < calc_eps || abs(D) < calc_eps )
	B=99999;
else
	if( abs(a(5)) < calc_eps )
		B=99999;
    else
        % BCD = lateral tire stiffness
        C_Fy=a(4)*sin(2*atan(Fz/a(5)))*(1-a(6)*abs(camber));
        B=C_Fy/(C*D);
	end
end
% E
E=a(7)*Fz+a(8);

% S = f(alpha)
S=alpha+a(9)*camber+a(10)*Fz+a(11);
Sv=(a(12)*Fz+a(13))*camber*Fz+a(13)*Fz+a(14);

% Resulting force
Fy=D*sin(C*atan(B*S-E*(B*S-atan(B*S))))+Sv;

== matlab function vehicle_dynamics_lib/Force elements/Spring-Damper/Semi Active/Semi-active force ==
  data: v_defl input size=1; f_out output size=1; f_in input size=1; d_s_max parameter
function f_out = semiact(v_defl,f_in,d_s_max)
%#eml

if( f_in * v_defl > 0 )
    f_out = sign(f_in)*min(d_s_max*abs(v_defl),abs(f_in));
else
    f_out = 0;
end

== matlab function vehicle_dynamics_lib/Force elements/Wheel forces & torques/Calculate tire forces ==
  data: pos input size=3; Ftire output size=3; M_resist output; vel input size=3; axle input size=3; whlvel input size=3; GND_DATA input; c parameter size=1; d parameter size=1; sx output; alpha output; r0 parameter
function [Ftire, M_resist, sx, alpha]  = tire_force(pos, vel, axle, whlvel, GND_DATA , c, d, r0)
%#eml

n = GND_DATA(2:4);    % Normal to ground
Z = GND_DATA(1);    % z-height of ground
v_thres = 1e-1; % Threshold of slip
alpha_thres = 1e-1; % Threshold for slip angle
mu = 1;          % road friciton coefficient
qsy1 = 0.01;    % rolling friction coefficient
V0 = 16.66;     % reference velocity [m/s]

%% Calculate normal force
defl_n = n.'*([0;0;pos(3)-Z]);
if defl_n > 0   % No forces if wheel doesn't touch ground
    Ftire = zeros(3,1);
    M_resist = 0;
    sx = 0;
    alpha = 0;
    return;
end

Fn = -c*defl_n; % Vertical force due to tire stiffness
vel_n = n.'*vel;  % velocity of contact point normal to ground

if vel_n < 0    % damper only generates force on contraction
    Fn=Fn-d*vel_n;  
end

%% Calculate slip & slip angle
fwd = cross(axle,n);        % forward direction vector
fwd_len = sqrt(fwd.'*fwd);
%if( fwd_len < 1e-6 )
%   wheel axle nearly orthogonal to ground normal   
%end
fwd = fwd/fwd_len;  % longitudinal unit vector

lat = cross(n,fwd);  % lateral unit vector

% x-Dir
vx = fwd.'*vel;
vsgn = sign(vx);
avx = abs(vx);
whlvel_x = fwd.'*whlvel;
awhlvel_x = abs(whlvel_x);
sx = avx/(awhlvel_x+v_thres);   % slip value

tmp = tanh(sqrt(avx*avx)/v_thres);
sx = tmp*tmp*sx;

% y-Dir
whlvel_y = lat.'*whlvel;
alpha = atan2(whlvel_y,awhlvel_x);  % slip angle
alphasgn = sign(alpha);
tmp = tanh(sqrt(whlvel_x*whlvel_x + whlvel_y*whlvel_y)/alpha_thres); % reduce alpha for low speeds
alpha = abs(alpha*tmp*tmp);

[Fx, Fy] = tire_force2(Fn, mu, sx, alpha);

Ftire = n*Fn - fwd*Fx*vsgn - lat*Fy*alphasgn;
fr = qsy1;
Fr = fr*Fn; % free rolling resistance
M_resist = -Fr*r0*tanh((whlvel_x-vx)/V0);
%% Calculate friction torque


function [Fx, Fy ] = tire_force2( Fz, mu, sx, alpha )
%TIRE_FORCE(Fz, mu, sx, alpha)
%   Calculation of lateral and longitudinal tire forces 
%       <Vehicle Dynamics, p. 48>
%   Fz - vertical load force in N
%   mu - road-tire friction coefficient
%   sx - longitudinal slip
%   alpha - slip angle
orgFz = Fz;
Fz = min(Fz,11e3);
Fz = max(2e3,Fz);

FzN = 3e3;

% Longitudinal parameters
dFx0N = 70e3;   dFx02N = 220e3;
sxMN = 0.16;    sxM2N = 0.12;
FxMN = 2.9e3;   FxM2N = 5.6e3;
sxSN = 0.5;     sxS2N = 0.5;
FxSN = 2.65e3;  FxS2N = 5.1e3;

% Lateral parameters
dFy0N = 72e3;   dFy02N = 130e3;
syMN = 0.18;    syM2N = 0.2;
FyMN = 2.85e3;  FyM2N = 5.4e3;
sySN = 0.5;     syS2N = 0.7;
FySN = 2.8e3;   FyS2N = 5.3e3;

% Interpolate parameters at Fz
intparam = load_interp22(Fz, FzN, [dFx0N;sxMN;FxMN;sxSN;FxSN; ...
	dFy0N;syMN;FyMN;sySN;FySN], [dFx02N;sxM2N;FxM2N;sxS2N;FxS2N; ...
    dFy02N;syM2N;FyM2N;syS2N;FyS2N])*mu;

dFx0 = intparam(1);
sxM = intparam(2);
FxM = intparam(3);
sxS = intparam(4);
FxS = intparam(5);

dFy0 = intparam(6);
syM = intparam(7);
FyM = intparam(8);
syS = intparam(9);
FyS = intparam(10);

%% Calculate longitudinal force
if( sx <= sxM )
    sigma = sx/sxM;
    Fx = (sxM*dFx0*sigma)/(1+sigma*(sigma+dFx0*sxM/FxM-2));
elseif( (sx <= sxS) && (sx > sxM ) )
    sigma = (sx-sxM)/(sxS-sxM);
    Fx = FxM-(FxM-FxS)*sigma^2*(3-2*sigma);
else
    Fx = FxS;
end

%% Calculate lateral force
if( alpha <= syM )
    sigma = alpha/syM;
    Fy = (syM*dFy0*sigma)/(1+sigma*(sigma+dFy0*syM/FyM-2));
elseif( (alpha <= syS) && (alpha > syM ) )
    sigma = (alpha-syM)/(syS-syM);
    Fy = FyM-(FyM-FyS)*sigma^2*(3-2*sigma);
else
    Fy = FyS;
end

Fx = min(Fx, orgFz*mu);
Fy = min(Fy, orgFz*mu);

% Decrease length of combined force vector, if bigger than max force
if( abs(FxM) < 1e-5 || abs(FyM) < 1e-5 )
    return;
end

nrmFx=Fx/FxM;
nrmFy=Fy/FyM;

% Calculate total vector size, but avoid the sqrt() for now
len=nrmFy*nrmFy+nrmFx*nrmFx;
%{ 
If the vector exceeds the friction circle (which, because
it is normalized, is a real circle with radius 1), the
forces are downsized accordingly to fit the circle.
Note that 1 squared is still 1 (len is still squared)
%}
if( len > 1 )
	% Get actual length (non-squared)
    len=sqrt(len);

    Fx=Fx/len;
    Fy=Fy/len;
end

function [ out ] = load_interp22( Fz, FzN, pN, p2N )
%LOAD_INTERP2 Summary of this function goes here
%   Detailed explanation goes here
pNtmp = zeros(length(pN),length(Fz));
for i=1:length(Fz)
    pNtmp(:,i) = pN;
end
out = pNtmp+(p2N-pN)*(Fz/FzN-1);

function [Fx, Fy] = kamm_circle(Fx, Fy)
%KAMM_CIRCLE
